simulink model "SISO_2"  (R2025b)
settings: Solver=VariableStepAuto  StartTime=0.0  StopTime=8  RelTol=1e-3
libraries: SignalEditorBlockLib x1
settings Model: Creator=Soochan Kim  LastModifiedBy=Soochan Kim

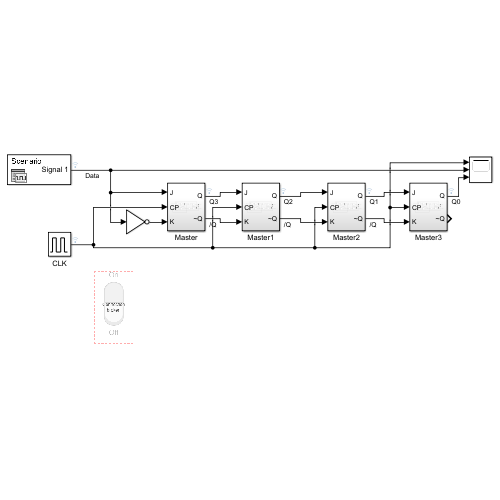
[thumbnail: Simulink's stored preview of the top-level diagram]
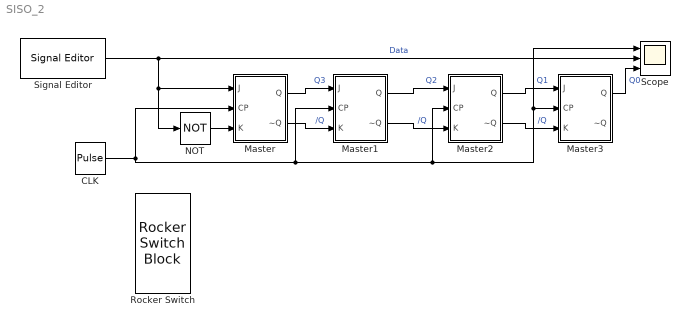
== system SISO_2 ==
  CLK : DiscretePulseGenerator  PulseType=Time based  Period=1  PulseWidth=50  PhaseDelay=0.5
  Master : Subsystem
  Master1 : Subsystem
  Master2 : Subsystem
  Master3 : Subsystem
  NOT : Logic  Operator=NOT  IconShape=distinctive  AllPortsSameDT=off  OutDataTypeStr=boolean
  Rocker Switch : RockerSwitchBlock
  Scope : Scope  NumInputPorts=3
      settings: ActiveDisplayYMinimum=-0.12499999999999997  ActiveDisplayYMaximum=1.125
  Signal Editor : SignalEditorBlockLib/Signal Editor  FileName=Signal1.mat  ActiveScenario=Scenario  ActiveSignal=Signal 1  IsBus=off  OutputBusObjectStr=Bus: BusObject  SampleTime=0  ZeroCross=off  OutputAfterFinalValue=Setting to zero  Unit=inherit  PreserveSignalName=on  ApplySigPropsToAllScenarios=on  ApplySigPropsToAllSignals=off  SignalPropertySource=Dialog parameters
  wires:
  Signal Editor/1 -> NOT/1, Master/1(J), Scope/2  "Data"
  CLK/1 -> Scope/1, Master3/2(CP), Master2/2(CP), Master1/2(CP), Master/2(CP)
  Master/1(Q) -> Master1/1(J)  "Q3"
  Master1/1(Q) -> Master2/1(J)  "Q2"
  Master2/1(Q) -> Master3/1(J)  "Q1"
  Master/2(~Q) -> Master1/3(K)  "/Q"
  Master1/2(~Q) -> Master2/3(K)  "/Q"
  Master2/2(~Q) -> Master3/3(K)  "/Q"
  NOT/1 -> Master/3(K)
  Master3/1(Q) -> Scope/3  "Q0"

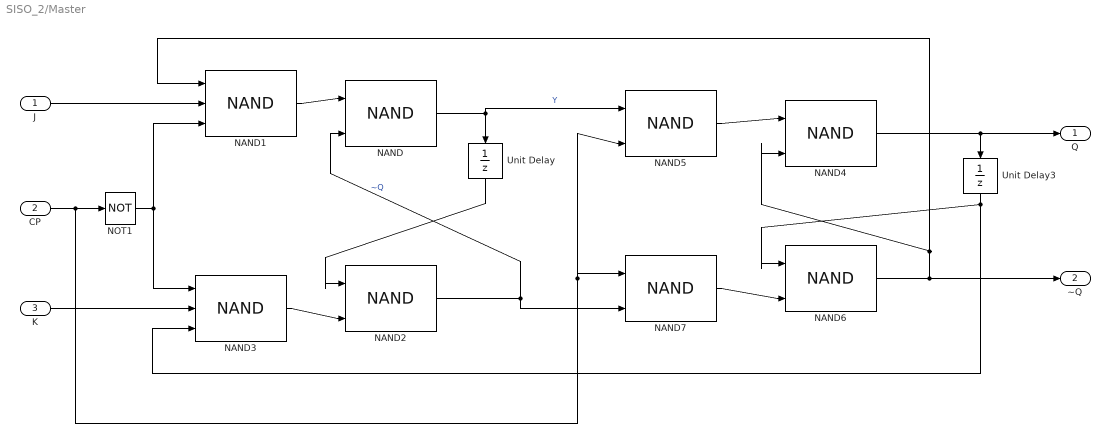
== system SISO_2/Master ==
  J : Inport
  CP : Inport  Port=2
  K : Inport  Port=3
  NAND{,2,4..7} (6 alike) : Logic  Operator=NAND  IconShape=distinctive  AllPortsSameDT=off  OutDataTypeStr=boolean
  NAND1 : Logic  Operator=NAND  Inputs=3  IconShape=distinctive  AllPortsSameDT=off  OutDataTypeStr=boolean
  NAND3 : Logic  Operator=NAND  Inputs=3  IconShape=distinctive  AllPortsSameDT=off  OutDataTypeStr=boolean
  NOT1 : Logic  Operator=NOT  IconShape=distinctive  AllPortsSameDT=off  OutDataTypeStr=boolean
  Unit Delay : UnitDelay  SampleTime=0.001  HasFrameUpgradeWarning=on
  Unit Delay3 : UnitDelay  SampleTime=-1  HasFrameUpgradeWarning=on
  Q : Outport
  ~Q : Outport  Port=2
  wires:
  NAND/1 -> Unit Delay/1, NAND5/1  "Y"
  NAND2/1 -> NAND/2, NAND7/2  "~Q"
  Unit Delay/1 -> NAND2/1
  K/1 -> NAND3/2
  NAND1/1 -> NAND/1
  NAND3/1 -> NAND2/2
  J/1 -> NAND1/2
  NAND6/1 -> ~Q/1, NAND1/1, NAND4/2
  Unit Delay3/1 -> NAND3/3, NAND6/1
  NAND5/1 -> NAND4/1
  NAND7/1 -> NAND6/2
  NAND4/1 -> Q/1, Unit Delay3/1
  CP/1 -> NAND5/2, NAND7/1, NOT1/1
  NOT1/1 -> NAND1/3, NAND3/1

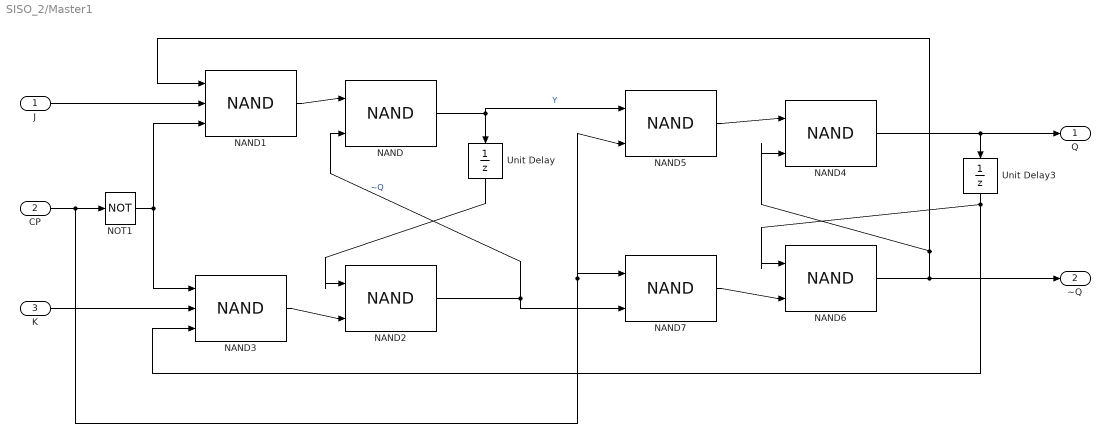
== system SISO_2/Master1 ==
  J : Inport
  CP : Inport  Port=2
  K : Inport  Port=3
  NAND{,2,4..7} (6 alike) : Logic  Operator=NAND  IconShape=distinctive  AllPortsSameDT=off  OutDataTypeStr=boolean
  NAND1 : Logic  Operator=NAND  Inputs=3  IconShape=distinctive  AllPortsSameDT=off  OutDataTypeStr=boolean
  NAND3 : Logic  Operator=NAND  Inputs=3  IconShape=distinctive  AllPortsSameDT=off  OutDataTypeStr=boolean
  NOT1 : Logic  Operator=NOT  IconShape=distinctive  AllPortsSameDT=off  OutDataTypeStr=boolean
  Unit Delay : UnitDelay  SampleTime=0.001  HasFrameUpgradeWarning=on
  Unit Delay3 : UnitDelay  SampleTime=-1  HasFrameUpgradeWarning=on
  Q : Outport
  ~Q : Outport  Port=2
  wires:
  NAND/1 -> Unit Delay/1, NAND5/1  "Y"
  NAND2/1 -> NAND/2, NAND7/2  "~Q"
  Unit Delay/1 -> NAND2/1
  K/1 -> NAND3/2
  NAND1/1 -> NAND/1
  NAND3/1 -> NAND2/2
  J/1 -> NAND1/2
  NAND6/1 -> ~Q/1, NAND1/1, NAND4/2
  Unit Delay3/1 -> NAND3/3, NAND6/1
  NAND5/1 -> NAND4/1
  NAND7/1 -> NAND6/2
  NAND4/1 -> Q/1, Unit Delay3/1
  CP/1 -> NAND5/2, NAND7/1, NOT1/1
  NOT1/1 -> NAND1/3, NAND3/1

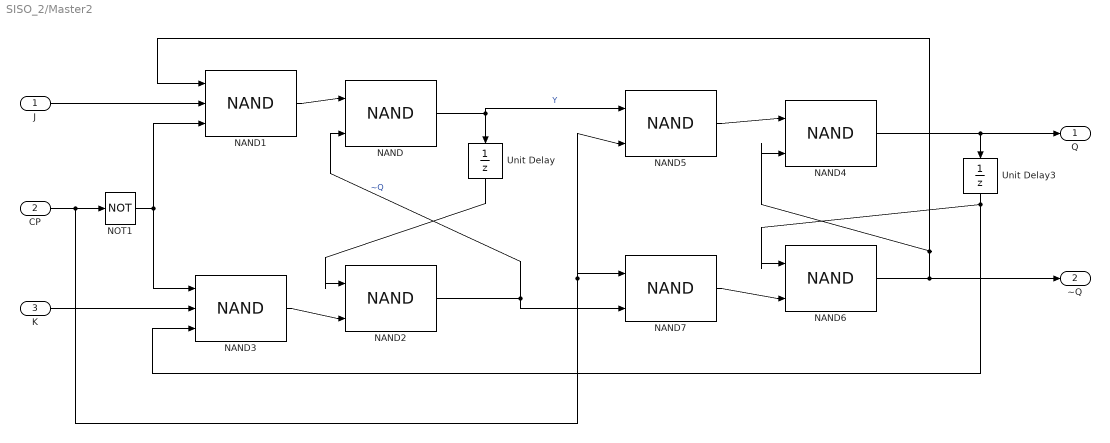
== system SISO_2/Master2 ==
  J : Inport
  CP : Inport  Port=2
  K : Inport  Port=3
  NAND{,2,4..7} (6 alike) : Logic  Operator=NAND  IconShape=distinctive  AllPortsSameDT=off  OutDataTypeStr=boolean
  NAND1 : Logic  Operator=NAND  Inputs=3  IconShape=distinctive  AllPortsSameDT=off  OutDataTypeStr=boolean
  NAND3 : Logic  Operator=NAND  Inputs=3  IconShape=distinctive  AllPortsSameDT=off  OutDataTypeStr=boolean
  NOT1 : Logic  Operator=NOT  IconShape=distinctive  AllPortsSameDT=off  OutDataTypeStr=boolean
  Unit Delay : UnitDelay  SampleTime=0.001  HasFrameUpgradeWarning=on
  Unit Delay3 : UnitDelay  SampleTime=-1  HasFrameUpgradeWarning=on
  Q : Outport
  ~Q : Outport  Port=2
  wires:
  NAND/1 -> Unit Delay/1, NAND5/1  "Y"
  NAND2/1 -> NAND/2, NAND7/2  "~Q"
  Unit Delay/1 -> NAND2/1
  K/1 -> NAND3/2
  NAND1/1 -> NAND/1
  NAND3/1 -> NAND2/2
  J/1 -> NAND1/2
  NAND6/1 -> ~Q/1, NAND1/1, NAND4/2
  Unit Delay3/1 -> NAND3/3, NAND6/1
  NAND5/1 -> NAND4/1
  NAND7/1 -> NAND6/2
  NAND4/1 -> Q/1, Unit Delay3/1
  CP/1 -> NAND5/2, NAND7/1, NOT1/1
  NOT1/1 -> NAND1/3, NAND3/1

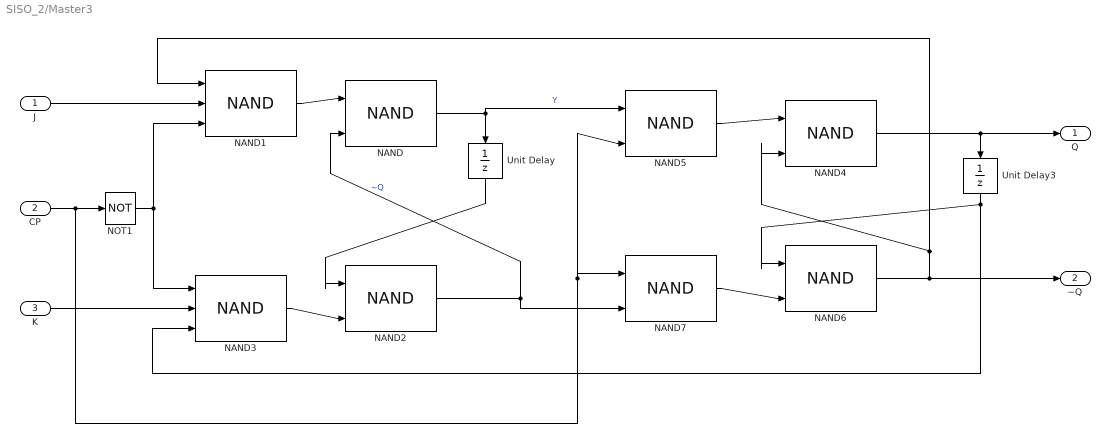
== system SISO_2/Master3 ==
  J : Inport
  CP : Inport  Port=2
  K : Inport  Port=3
  NAND{,2,4..7} (6 alike) : Logic  Operator=NAND  IconShape=distinctive  AllPortsSameDT=off  OutDataTypeStr=boolean
  NAND1 : Logic  Operator=NAND  Inputs=3  IconShape=distinctive  AllPortsSameDT=off  OutDataTypeStr=boolean
  NAND3 : Logic  Operator=NAND  Inputs=3  IconShape=distinctive  AllPortsSameDT=off  OutDataTypeStr=boolean
  NOT1 : Logic  Operator=NOT  IconShape=distinctive  AllPortsSameDT=off  OutDataTypeStr=boolean
  Unit Delay : UnitDelay  SampleTime=0.001  HasFrameUpgradeWarning=on
  Unit Delay3 : UnitDelay  SampleTime=-1  HasFrameUpgradeWarning=on
  Q : Outport
  ~Q : Outport  Port=2
  wires:
  NAND/1 -> Unit Delay/1, NAND5/1  "Y"
  NAND2/1 -> NAND/2, NAND7/2  "~Q"
  Unit Delay/1 -> NAND2/1
  K/1 -> NAND3/2
  NAND1/1 -> NAND/1
  NAND3/1 -> NAND2/2
  J/1 -> NAND1/2
  NAND6/1 -> ~Q/1, NAND1/1, NAND4/2
  Unit Delay3/1 -> NAND3/3, NAND6/1
  NAND5/1 -> NAND4/1
  NAND7/1 -> NAND6/2
  NAND4/1 -> Q/1, Unit Delay3/1
  CP/1 -> NAND5/2, NAND7/1, NOT1/1
  NOT1/1 -> NAND1/3, NAND3/1
